simulink model "testsim2"  (R2022b)
settings: Solver=ode4  StartTime=0.0  StopTime=simTime  FixedStep=dt  RelTol=1e-3
InitFcn:
  | parameters;
undefined symbols (not defined in the file or in its folder): delta_v1, delta_v2, delta_v3, delv4, initial_position, initial_velocity, JDlaunch, km, mu_earth, mu_moon, s, t4, T_injec, T_trans
libraries: aerolibcelestial x1
settings Model: Creator=dongmin  LastModifiedBy=dongmin

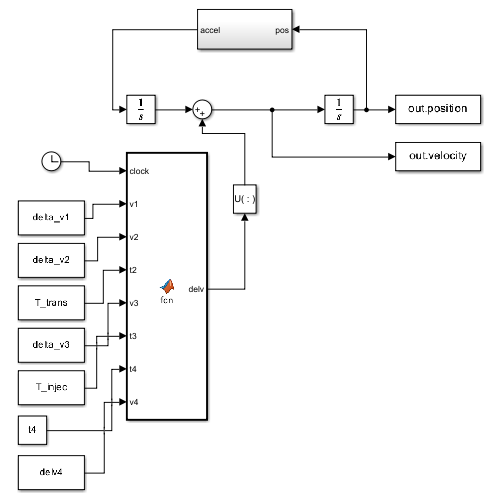
[thumbnail: Simulink's stored preview of the top-level diagram]
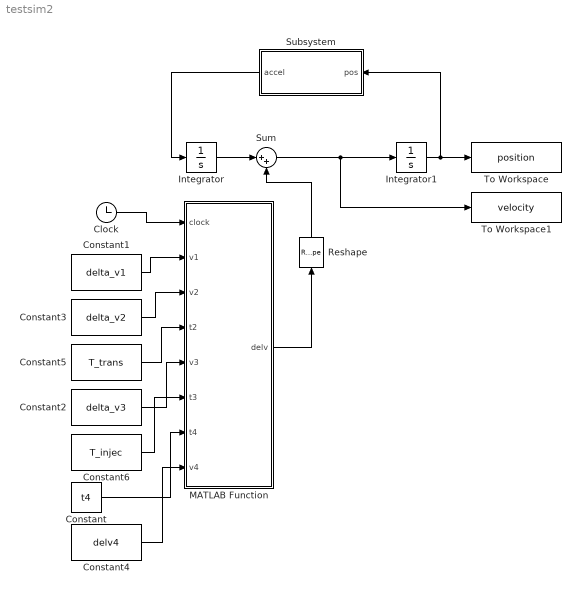
== system testsim2 ==
  Clock : Clock
  Constant : Constant  Value=t4
  Constant1 : Constant  Value=delta_v1
  Constant2 : Constant  Value=delta_v3
  Constant3 : Constant  Value=delta_v2
  Constant4 : Constant  Value=delv4
  Constant5 : Constant  Value=T_trans
  Constant6 : Constant  Value=T_injec
  Integrator : Integrator  InitialCondition=initial_velocity
  Integrator1 : Integrator  InitialCondition=initial_position
  MATLAB Function : MATLAB Function  TreatAsAtomicUnit=on
  Reshape : Reshape
  Subsystem : Subsystem
  Sum : Sum  Inputs=|++
  To Workspace : ToWorkspace  VariableName=position  SaveFormat=Timeseries  SampleTime=-1
  To Workspace1 : ToWorkspace  VariableName=velocity  SaveFormat=Timeseries  SampleTime=-1
  wires:
  Integrator1/1 -> Subsystem/1(pos), To Workspace/1
  Integrator/1 -> Sum/1
  Sum/1 -> To Workspace1/1, Integrator1/1
  Constant6/1 -> MATLAB Function/6(t3)
  Constant2/1 -> MATLAB Function/5(v3)
  Constant5/1 -> MATLAB Function/4(t2)
  Constant3/1 -> MATLAB Function/3(v2)
  Constant1/1 -> MATLAB Function/2(v1)
  Clock/1 -> MATLAB Function/1(clock)
  MATLAB Function/1(delv) -> Reshape/1
  Reshape/1 -> Sum/2
  Subsystem/1(accel) -> Integrator/1
  Constant/1 -> MATLAB Function/7(t4)
  Constant4/1 -> MATLAB Function/8(v4)

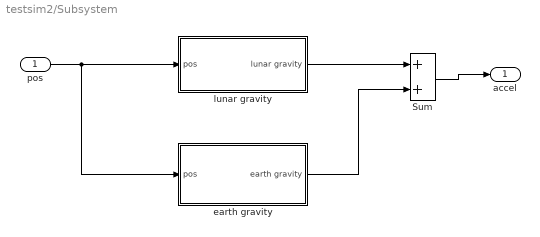
== system testsim2/Subsystem ==
  pos : Inport
  Sum : Sum
  earth gravity : Subsystem
  lunar gravity : Subsystem
  accel : Outport
  wires:
  pos/1 -> earth gravity/1(pos), lunar gravity/1(pos)
  lunar gravity/1(lunar gravity) -> Sum/1
  earth gravity/1(earth gravity) -> Sum/2
  Sum/1 -> accel/1

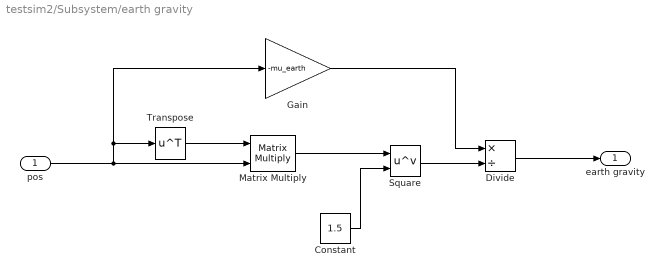
== system testsim2/Subsystem/earth gravity ==
  pos : Inport
  Constant : Constant  Value=1.5
  Divide : Product  Inputs=*/
  Gain : Gain  Gain=-mu_earth
  Matrix Multiply : Product  Multiplication=Matrix(*)
  Square : Math  Operator=pow
  Transpose : Math  Operator=transpose
  earth gravity : Outport
  wires:
  Gain/1 -> Divide/1
  Matrix Multiply/1 -> Square/1
  pos/1 -> Gain/1, Transpose/1, Matrix Multiply/2
  Transpose/1 -> Matrix Multiply/1
  Divide/1 -> earth gravity/1
  Square/1 -> Divide/2
  Constant/1 -> Square/2

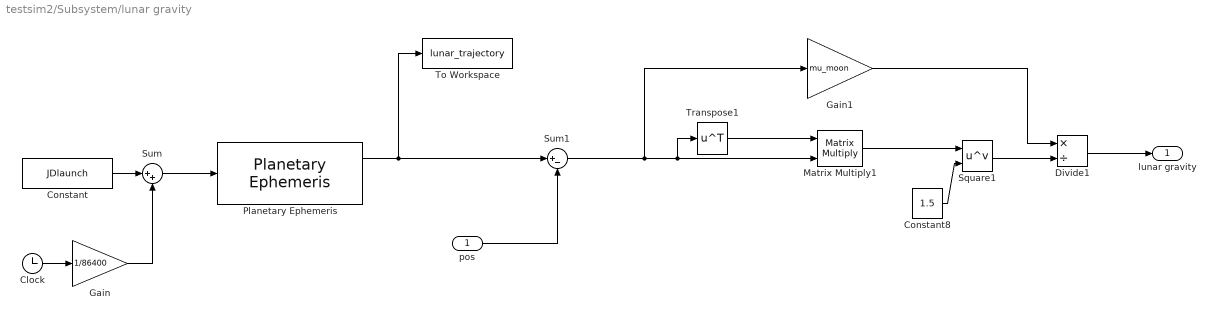
== system testsim2/Subsystem/lunar gravity ==
  pos : Inport
  Clock : Clock
  Constant : Constant  Value=JDlaunch
  Constant8 : Constant  Value=1.5
  Divide1 : Product  Inputs=*/
  Gain : Gain  Gain=1/86400
  Gain1 : Gain  Gain=mu_moon
  Matrix Multiply1 : Product  Multiplication=Matrix(*)
  Planetary Ephemeris : aerolibcelestial/Planetary Ephemeris  kmflag=km,km/s  epochflag=Julian date  de=DE405  nCenter=Earth  nTarget=Moon  errorflag=Error  velflag=on
  Square1 : Math  Operator=pow
  Sum : Sum  Inputs=|++
  Sum1 : Sum  Inputs=|+-
  To Workspace : ToWorkspace  VariableName=lunar_trajectory  SaveFormat=Timeseries  SampleTime=-1
  Transpose1 : Math  Operator=transpose
  lunar gravity : Outport
  wires:
  Sum1/1 -> Transpose1/1, Matrix Multiply1/2, Gain1/1
  Matrix Multiply1/1 -> Square1/1
  Gain1/1 -> Divide1/1
  Divide1/1 -> lunar gravity/1
  Transpose1/1 -> Matrix Multiply1/1
  Constant8/1 -> Square1/2
  Planetary Ephemeris/1 -> Sum1/1, To Workspace/1
  Square1/1 -> Divide1/2
  pos/1 -> Sum1/2
  Constant/1 -> Sum/1
  Clock/1 -> Gain/1
  Gain/1 -> Sum/2
  Sum/1 -> Planetary Ephemeris/1

== matlab function testsim2/MATLAB Function ==
  data: clock input; delv output; v1 input; v2 input; t2 input; v3 input; t3 input; t4 input; v4 input
function delv = fcn(clock,v1,v2,t2,v3,t3,t4,v4)

delv = v1;

if clock > t2+t3+t4
    delv = v1+v2+v3+v4;
elseif clock > t2+t3
    delv = v1+v2+v3;
elseif clock > t2
    delv = v1+v2;

end
